simulink model "ForwardVehicleSensorFusion"  (R2022b)
settings: Solver=FixedStepAuto  StartTime=0.0  StopTime=Inf  RelTol=1e-3  SampleTimeConstraint=STIndependent
model workspace (MAT data in the model file):
  numDetsPerCluster = 10
  numDetsPerSensor = 36
  numEvents = 5
  numTracksPerCluster = 10
undefined symbols (not defined in the file): assigThresh, Epsilon, M, MinNumPoints, N, P, R
libraries: trackingutilitieslib x1, motalgorithmslib x1
settings Model: Creator=The MathWorks, Inc.  LastModifiedBy=The MathWorks, Inc.
settings SolverCC: AlgebraicLoopSolver=TrustRegion  MaxZcPerStep=1
settings DataIOCC: SaveOutput=off  SaveTime=off  ReturnWorkspaceOutputs=off
settings OptimizationCC: DefaultParameterBehavior=Inlined  InlineInvariantSignals=on  EnhancedBackFolding=on  PassReuseOutputArgsAs=Individual arguments  ZeroExternalMemoryAtStartup=off  ZeroInternalMemoryAtStartup=off  EfficientFloat2IntCast=on  OptimizeBlockOrder=speed  DifferentSizesBufferReuse=on  OptimizationCustomize=off  EfficientTunableParamExpr=on
settings DebuggingCC: ParameterPrecisionLossMsg=none  ParameterTunabilityLossMsg=error  UnconnectedInputMsg=warning  UnconnectedOutputMsg=warning  UnconnectedLineMsg=warning  PregeneratedLibrarySubsystemCodeDiagnostic=none  SFMachineParentedDataDiag=warning  ArithmeticOperatorsInVariantConditions=warning
settings HardwareCC: ProdLongLongMode=on
settings ModelReferenceCC: EnableRefExpFcnMdlSchedulingChecks=on
settings SFSimCC: SimUseLocalCustomCode=off  SimTargetLang=C++
settings RTWCC: Description=Embedded Coder  SystemTargetFile=ert.tlc  GenCodeOnly=on  TemplateMakefile=ert_default_tmf  RTWVerbose=off  RTWUseLocalCustomCode=off  BuildConfiguration=Faster Runs  TargetLang=C++  DLArmComputeVersion=19.05
settings CodeAppCC: ForceParamTrailComments=on  IgnoreCustomStorageClasses=off  MaxIdLength=256  OperatorAnnotations=on  SimulinkDataObjDesc=on  SFDataObjDesc=on  CustomSymbolStrGlobalVar=fvsf$N$M  CustomSymbolStrType=fvsf$N$M_T  CustomSymbolStrFcn=fvsf$N$M$F  CustomSymbolStrMacro=fvsf$N$M  InsertBlockDesc=on
settings ERTTargetCC: TargetLangStandard=C++03 (ISO)  GenerateSampleERTMain=on  CombineSignalStateStructs=on  CodeInterfacePackaging=C++ class  SupportVariableSizeSignals=on  InlinedParameterPlacement=NonHierarchical  RootIOFormat=Structure reference  ERTCustomFileTemplate=example_file_process.tlc
settings ConfigComp: CovScope=ReferencedModels  CovIncludeTopModel=off

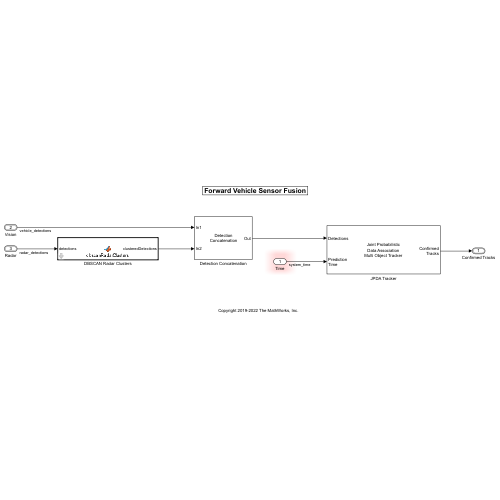
[thumbnail: Simulink's stored preview of the top-level diagram]
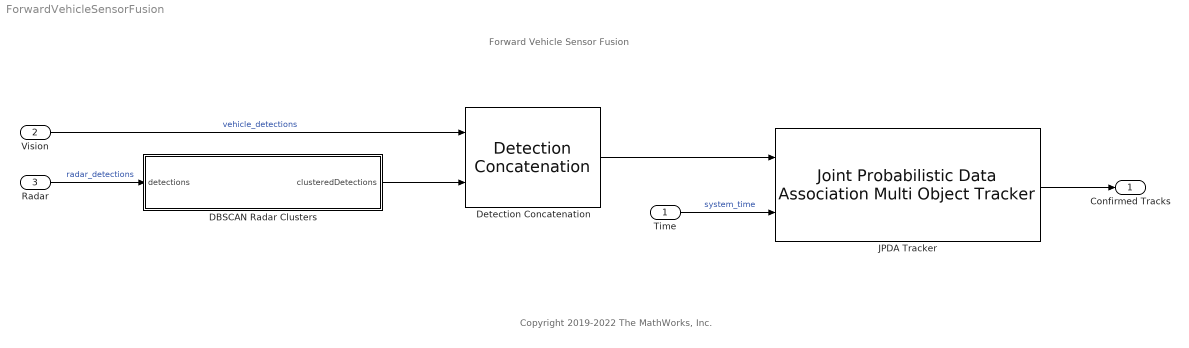
== system ForwardVehicleSensorFusion ==
  note: Forward Vehicle Sensor Fusion
  note: Copyright 2019-2022 The MathWorks, Inc.
  Time : Inport  OutDataTypeStr=TimeDataType
  Vision : Inport  Port=2  OutDataTypeStr=Bus: BusVision  BusOutputAsStruct=on
  Radar : Inport  Port=3  OutDataTypeStr=Bus: BusRadar  BusOutputAsStruct=on
  DBSCAN Radar Clusters : MATLAB Function  TreatAsAtomicUnit=on  mask{azRes=0.8, rrRes=1, rRes=1, epsilon=Epsilon, minNumPts=MinNumPoints}
      mask prompts: azRes "Azimuthal Resolution"; rrRes "Range Rate Resolution"; rRes "Range Resolution"; minNumPts "Minimum Number of Points"
  Detection Concatenation : trackingutilitieslib/Detection Concatenation  NumInputs=2  BusNameSource=Property  BusName=BusDetectionConcatenation1  SimulateUsing=Interpreted execution
  JPDA Tracker : motalgorithmslib/Joint Probabilistic Data Association Multi Object Tracker  TrackerIndex=uint32( 0 )  FilterInitializationFcn=helperInitFilter  MaxNumEvents=numEvents  EventGenerationFcn=jpdaEvents  MaxNumTracks=numTracks  MaxNumSensors=numSensors  TimeTolerance=1e-5  OOSMHandling=Terminate  MaxNumOOSMSteps=3  StateParametersSimulink=struct  HasStateParametersInput=off  EnableMemoryManagement=on  SimulateUsing=Interpreted execution  AssignmentThreshold=[ 1, Inf ] * assigThresh  InitializationThreshold=0  DetectionProbability=0.9  ClutterDensity=1e-06  TrackLogic=History  pHistoryConfThreshold=[ M, N ]  pHistoryDelThreshold=[ P, R ]  pIntegratedConfThreshold=0.95  pIntegratedDelThreshold=0.1  HitMissThreshold=0.5  NewTargetDensity=1e-5  DeathRate=0.01  TimeInputSource=Input port  HasCostMatrixInput=off  HasDetectableTrackIDsInput=off  TentativeTracksOutputPort=off  AllTracksOutputPort=off  InfoOutputPort=off  BusNameSource=Property  BusName=BusTrackerJPDA  BusName2Source=Auto  BusName2=BusTrackerInfo  MaxNumDetectionsPerSensor=numDetsPerSensor  MaxNumDetectionsPerCluster=numDetsPerCluster  MaxNumTracksPerCluster=numTracksPerCluster  ClusterViolationHandling=Terminate
  Confirmed Tracks : Outport  OutDataTypeStr=Bus: BusTrackerJPDA  BusOutputAsStruct=on
  wires:
  Radar/1 -> DBSCAN Radar Clusters/1(detections)  "radar_detections"
  Vision/1 -> Detection Concatenation/1  "vehicle_detections"
  JPDA Tracker/1 -> Confirmed Tracks/1
  Detection Concatenation/1 -> JPDA Tracker/1
  DBSCAN Radar Clusters/1(clusteredDetections) -> Detection Concatenation/2
  Time/1 -> JPDA Tracker/2  "system_time"

== matlab function ForwardVehicleSensorFusion/DBSCAN Radar Clusters ==
  data: detections input; clusteredDetections output Bus: BusRadar; azRes parameter; rrRes parameter; rRes parameter; epsilon parameter; minNumPts parameter
function clusteredDetections = dbscanRadarClusters(detections, azRes, rrRes, rRes, epsilon, minNumPts)

if detections.NumDetections == 0
    clusteredDetections = detections;
    return;
end

azRes     = cast(azRes, 'like', detections.Detections(1).Time);
rrRes     = cast(rrRes, 'like', detections.Detections(1).Time);
epsilon   = cast(epsilon, 'like', detections.Detections(1).Time);
minNumPts = cast(minNumPts, 'like', detections.Detections(1).Time);

scaleMatrix = diag(1./[azRes rRes rrRes]);
scaleInverseMatrix = diag([azRes rRes rrRes]);

inDets = detections.Detections(1:detections.NumDetections);

% Pre-process measurements in az, el, range to account for non-linearity
for i = 1:numel(inDets)
    inDets(i).Measurement = scaleMatrix*inDets(i).Measurement;
    inDets(i).MeasurementNoise = scaleMatrix*inDets(i).MeasurementNoise*scaleMatrix;
end 

clusterIdx = partitionDetections(inDets,epsilon,minNumPts,'Algorithm','DBSCAN','Distance','Euclidean');
clusteredDets = mergeDetections(inDets,clusterIdx);

% Post-process the clusters to account for transformation
for i = 1:numel(clusteredDets)
    clusteredDets(i).Measurement = scaleInverseMatrix*clusteredDets(i).Measurement;
    clusteredDets(i).MeasurementNoise = scaleInverseMatrix*clusteredDets(i).MeasurementNoise*scaleInverseMatrix;
end

clusteredDetections = coder.nullcopy(detections);
clusteredDetections.Detections(1:numel(clusteredDets)) = clusteredDets;
clusteredDetections.NumDetections(1) = numel(clusteredDets);
